simulink model "qpsk_phase_de"  (R2016b)
settings: Solver=VariableStepAuto  StartTime=0.0  StopTime=(12+8+175)*8*2-1  RelTol=1e-3  EnableMultiTasking=on
values from neighbouring files (symbols this model uses):
  K1 = K1/(K0*Kp)    [kfunc.m]
  K2 = K2/(K0*Kp)    [kfunc.m]
undefined symbols (not defined in the file or in its folder): jsin, rcosine
libraries: dspstat3 x1
settings Model: Creator=coltmt  LastModifiedBy=colttom
settings DataIOCC: LimitDataPoints=on
settings OptimizationCC: LifeSpan=inf
settings DebuggingCC: AllowSymbolicDim=off  SFUnexpectedBacktrackingDiag=warning  SFNoUnconditionalDefaultTransitionDiag=warning  SFExecutionAtInitializationDiag=none
settings ModelReferenceCC: PropagateSignalLabelsOutOfModel=off
settings GRTTargetCC: TargetLangStandard=C89/C90 (ANSI)
settings ConfigComp: CovMetricSettings=dw  CovHtmlReporting=on  CovSaveCumulativeToWorkspaceVar=on  CovSaveSingleToWorkspaceVar=on  CovExternalEMLEnable=off

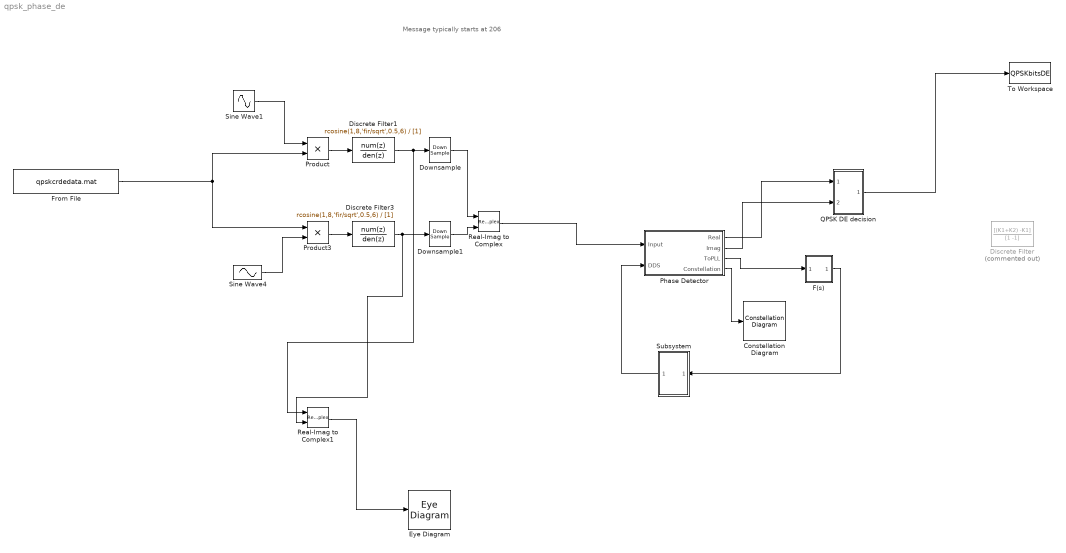
== system qpsk_phase_de ==
  note: Message typically starts at 206
  Constellation Diagram : ConstellationDiagram
  Discrete Filter : DiscreteFilter  Commented=on  Numerator=[(K1+K2) -K1]  Denominator=[1 -1]
  Discrete Filter1 : DiscreteFilter  Numerator=rcosine(1,8,'fir/sqrt',0.5,6)  Denominator=[1]
  Discrete Filter3 : DiscreteFilter  Numerator=rcosine(1,8,'fir/sqrt',0.5,6)  Denominator=[1]
  Downsample : DownSample  N=8  InputProcessing=Inherited (this choice will be removed - see release notes)  RateOptions=Allow multirate processing
  Downsample1 : DownSample  N=8  InputProcessing=Inherited (this choice will be removed - see release notes)  RateOptions=Allow multirate processing
  Eye Diagram : EyeDiagram
  F(s) : Subsystem
  From File : FromFile  FileName=qpskcrdedata.mat
  Phase Detector : Subsystem
  Product : Product
  Product3 : Product
  QPSK DE decision : Subsystem
  Real-Imag to Complex : RealImagToComplex
  Real-Imag to Complex1 : RealImagToComplex
  Sine Wave1 : Sin  Amplitude=sqrt(2)  Frequency=.3*2*pi  Phase=pi/2  SampleTime=1
  Sine Wave4 : Sin  Amplitude=-sqrt(2)  Frequency=.3*2*pi  SampleTime=1
  Subsystem : Subsystem
  To Workspace : ToWorkspace  VariableName=QPSKbitsDE  SampleTime=-1
  wires:
  Sine Wave1/1 -> Product/1
  Sine Wave4/1 -> Product3/2
  Product/1 -> Discrete Filter1/1
  Product3/1 -> Discrete Filter3/1
  Discrete Filter1/1 -> Real-Imag to Complex1/1, Downsample/1
  From File/1 -> Product/2, Product3/1
  Discrete Filter3/1 -> Real-Imag to Complex1/2, Downsample1/1
  Real-Imag to Complex1/1 -> Eye Diagram/1
  Downsample/1 -> Real-Imag to Complex/1
  Downsample1/1 -> Real-Imag to Complex/2
  F(s)/1(Out1) -> Subsystem/1(In1)
  Real-Imag to Complex/1 -> Phase Detector/1(Input)
  Subsystem/1(Out1) -> Phase Detector/2(DDS)
  Phase Detector/3(ToPLL) -> F(s)/1(In1)
  Phase Detector/4(Constellation) -> Constellation Diagram/1
  Phase Detector/1(Real) -> QPSK DE decision/1(In1)
  Phase Detector/2(Imag) -> QPSK DE decision/2(In2)
  QPSK DE decision/1(Out1) -> To Workspace/1

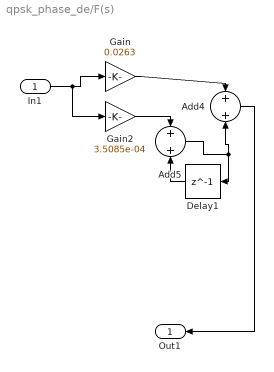
== system qpsk_phase_de/F(s) ==
  In1 : Inport
  Add4 : Sum
  Add5 : Sum
  Delay1 : Delay  DelayLength=1
  Gain : Gain  Gain=0.0263
  Gain2 : Gain  Gain=3.5085e-04
  Out1 : Outport
  wires:
  Gain/1 -> Add4/1
  Delay1/1 -> Add5/2
  Add5/1 -> Delay1/1, Add4/2
  Gain2/1 -> Add5/1
  Add4/1 -> Out1/1
  In1/1 -> Gain2/1, Gain/1

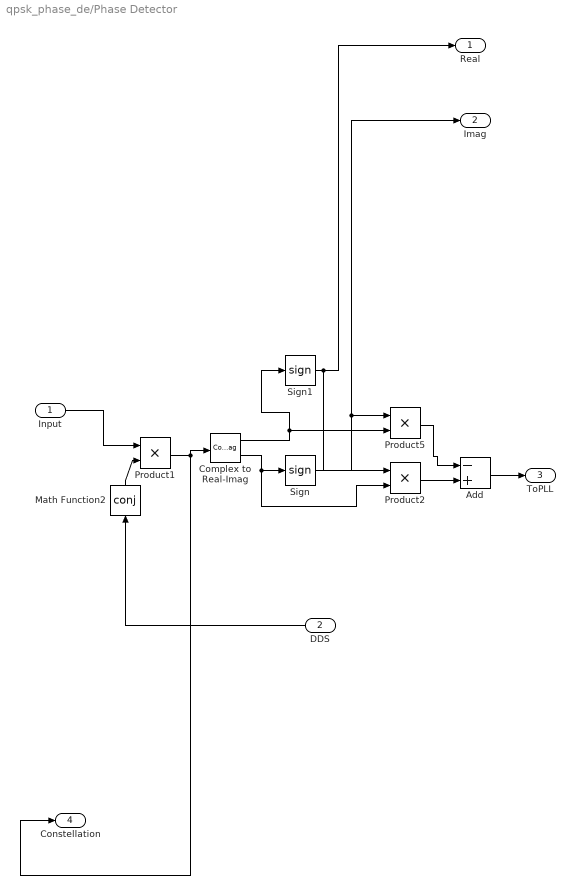
== system qpsk_phase_de/Phase Detector ==
  Input : Inport
  DDS : Inport  Port=2
  Add : Sum  Inputs=-+
  Complex to Real-Imag : ComplexToRealImag
  Math Function2 : Math  Operator=conj  SaturateOnIntegerOverflow=on
  Product1 : Product
  Product2 : Product
  Product5 : Product
  Sign : Signum
  Sign1 : Signum
  Real : Outport
  Imag : Outport  Port=2
  ToPLL : Outport  Port=3
  Constellation : Outport  Port=4
  wires:
  Add/1 -> ToPLL/1
  DDS/1 -> Math Function2/1
  Complex to Real-Imag/2 -> Product2/2, Sign/1
  Math Function2/1 -> Product1/2
  Product5/1 -> Add/1
  Product2/1 -> Add/2
  Input/1 -> Product1/1
  Complex to Real-Imag/1 -> Sign1/1, Product5/2
  Sign1/1 -> Real/1, Product2/1
  Sign/1 -> Imag/1, Product5/1
  Product1/1 -> Constellation/1, Complex to Real-Imag/1

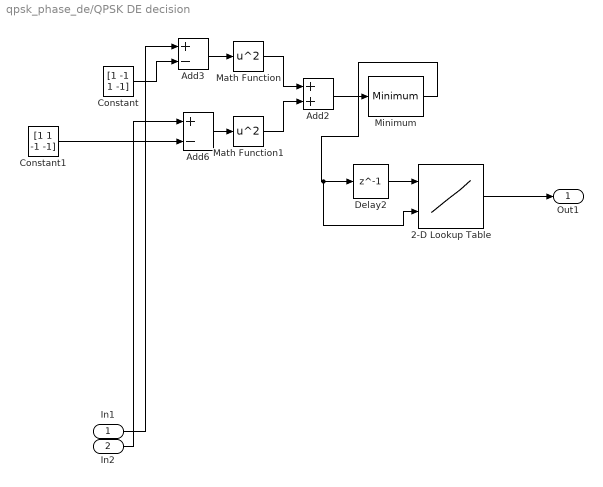
== system qpsk_phase_de/QPSK DE decision ==
  In1 : Inport
  In2 : Inport  Port=2
  2-D Lookup Table : Lookup_n-D  BreakpointsForDimension1=[0:3]  BreakpointsForDimension2=[0:3]  Table=[0 1 2 3; 2 0 3 1; 1 3 0 2;3 2 1 0]  InternalRulePriority=Speed  RndMeth=Simplest  InputSameDT=on
  Add2 : Sum
  Add3 : Sum  Inputs=+-
  Add6 : Sum  Inputs=+-
  Constant : Constant  Value=[1 -1 1 -1]
  Constant1 : Constant  Value=[1 1 -1 -1]
  Delay2 : Delay  DelayLength=1
  Math Function : Math  Operator=square  SaturateOnIntegerOverflow=on
  Math Function1 : Math  Operator=square  SaturateOnIntegerOverflow=on
  Minimum : dspstat3/Minimum  operation=minimum  fcn=Index  indexBase=Zero  operateOver=Each column  Dimension=1  InputProcessing=Columns as channels (frame based)  reset=None  roiEnable=off  roiType=Rectangles  roiPortion=Entire ROI  roiOutput=Individual statistics for each ROI  roiFlag=off  roundingMode=Floor  overflowMode=off
  Out1 : Outport
  wires:
  In1/1 -> Add3/1
  In2/1 -> Add6/1
  Math Function/1 -> Add2/1
  Math Function1/1 -> Add2/2
  Add3/1 -> Math Function/1
  Add6/1 -> Math Function1/1
  Constant/1 -> Add3/2
  Constant1/1 -> Add6/2
  Add2/1 -> Minimum/1
  Minimum/1 -> 2-D Lookup Table/2, Delay2/1
  2-D Lookup Table/1 -> Out1/1
  Delay2/1 -> 2-D Lookup Table/1

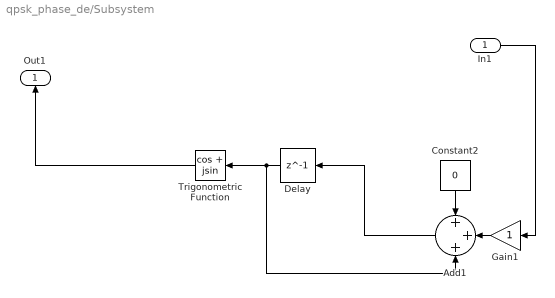
== system qpsk_phase_de/Subsystem ==
  In1 : Inport
  Add1 : Sum  Inputs=+++
  Constant2 : Constant  Value=0
  Delay : Delay  DelayLength=1
  Gain1 : Gain
  Trigonometric Function : Trigonometry  Operator=cos + jsin
  Out1 : Outport
  wires:
  In1/1 -> Gain1/1
  Constant2/1 -> Add1/1
  Add1/1 -> Delay/1
  Delay/1 -> Trigonometric Function/1, Add1/3
  Gain1/1 -> Add1/2
  Trigonometric Function/1 -> Out1/1
